simulink model "F16trim"  (R2013a)
settings: Solver=ode4  StartTime=0.0  StopTime=1  FixedStep=0.01  RelTol=1e-3
values from neighbouring files (symbols this model uses):
  airSpeed = 393.720000000000    (= 393.72)    [F16NolinearModelRemoveWindControlData_low.m]    (also in testdata.m)
  altitude = 9843    [F16Data.mat]    (also in F16LinmodTestData.m = trim_state(3); F16NolinearModelInitialData.m = trim_state(3); F16NolinearModelRemoveWindControlData_low.m; F16hi_7500_394_all.mat = 7500)
  b_ref = 9.144    [F16LinmodTestData.m]    (also in F16NolinearModelInitialData.m; F16NolinearModelRemoveWindControlData_low.m = 30; testdata.m = 30)
  beta = 0    [F16NolinearModelRemoveWindControlData_low.m]    (also in testdata.m)
  mass = 636.94*14.59428    (= 9295.6807032)    [F16LinmodTestData.m]    (also in F16NolinearModelInitialData.m; F16NolinearModelRemoveWindControlData_low.m = 636.94; testdata.m = 636.94)
  pqr = [0,0,0]    [F16NolinearModelRemoveWindControlData_low.m]    (also in testdata.m)
libraries: aerolibconvert2 x1, aerolibatmos2 x1, aerolibgravity2 x1, aerolibadyn x1
settings Model: Creator=Dai  LastModifiedBy=Dai

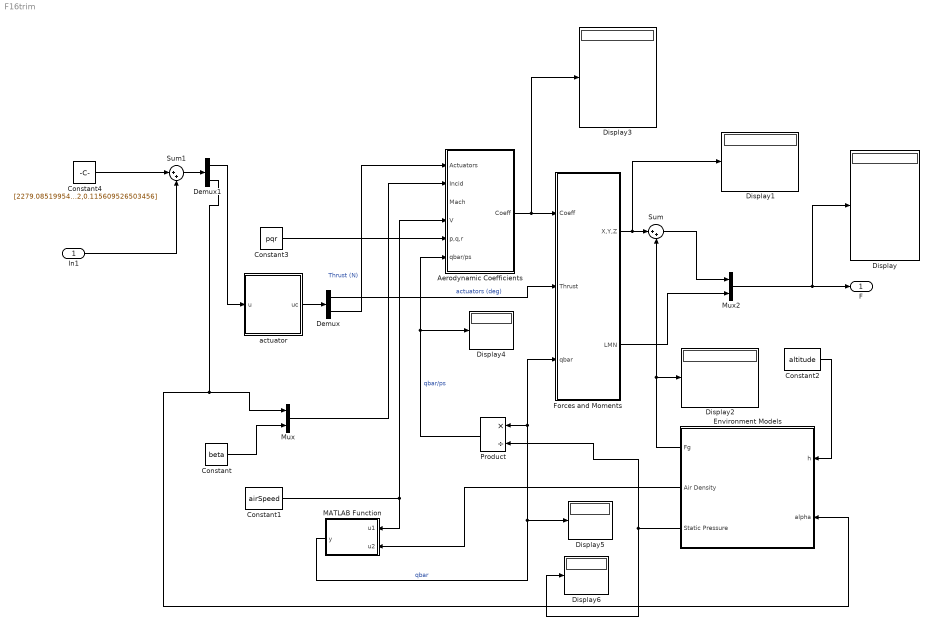
== system F16trim ==
  In1 : Inport  PortDimensions=5
  Aerodynamic Coefficients : Subsystem
  Constant : Constant  Value=beta
  Constant1 : Constant  Value=airSpeed
  Constant2 : Constant  Value=altitude
  Constant3 : Constant  Value=pqr
  Constant4 : Constant  Value=[2279.08519954656,-2.979731649,0.00874607850103852,0.0680302158182712,0.115609526503456]
  Demux : Demux  Outputs=2
  Demux1 : Demux  Outputs=[4,1]
  Display{,1..6} (7 alike) : Display
      Display settings: Decimation=6
      Display1 settings: Decimation=3
      Display2 settings: Decimation=3
      Display3 settings: Decimation=6
  Environment Models : Subsystem
  Forces and Moments : Subsystem
  MATLAB Function : MATLAB Function  TreatAsAtomicUnit=on
  Mux : Mux  Inputs=2
  Mux2 : Mux  Inputs=2
  Product : Product  Inputs=*/  SaturateOnIntegerOverflow=on  InputSameDT=on  OutDataTypeStr=Inherit: Same as first input
  Sum : Sum  Inputs=|++  SaturateOnIntegerOverflow=on  InputSameDT=on  OutDataTypeStr=Inherit: Same as first input
  Sum1 : Sum  Inputs=|++
  actuator : Subsystem
  F : Outport  PortDimensions=6
  wires:
  Aerodynamic Coefficients/1(Coeff) -> Display3/1, Forces and Moments/1(Coeff)
  Environment Models/2(Air Density) -> MATLAB Function/2(u2)
  Forces and Moments/2(LMN) -> Mux2/2
  MATLAB Function/1(y) -> Forces and Moments/3(qbar), Product/1, Display5/1  "qbar"
  Forces and Moments/1(X,Y,Z) -> Display1/1, Sum/1
  Environment Models/1(Fg) -> Display2/1, Sum/2
  Environment Models/3(Static Pressure) -> Display6/1, Product/2
  Product/1 -> Aerodynamic Coefficients/6(qbar/ps), Display4/1  "qbar/ps"
  actuator/1(uc) -> Demux/1
  Demux/1 -> Forces and Moments/2(Thrust)  "actuators (deg)"
  Demux/2 -> Aerodynamic Coefficients/1(Actuators)  "Thrust (N)"
  Demux1/2 -> Environment Models/2(alpha), Mux/1
  Constant/1 -> Mux/2
  Mux/1 -> Aerodynamic Coefficients/2(Incid)
  Constant1/1 -> MATLAB Function/1(u1), Aerodynamic Coefficients/4(V)
  Constant2/1 -> Environment Models/1(h)
  Constant3/1 -> Aerodynamic Coefficients/5(p,q,r)
  Demux1/1 -> actuator/1(u)
  Mux2/1 -> Display/1, F/1
  Constant4/1 -> Sum1/1
  Sum1/1 -> Demux1/1
  Sum/1 -> Mux2/1
  In1/1 -> Sum1/2

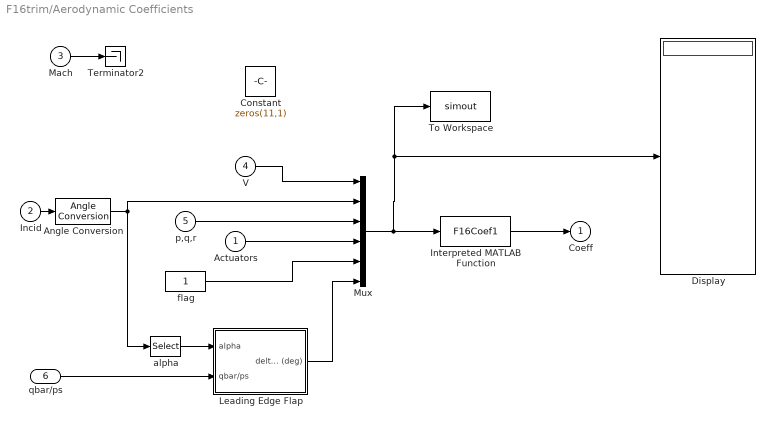
== system F16trim/Aerodynamic Coefficients ==
  Actuators : Inport
  Incid : Inport  Port=2
  Mach : Inport  Port=3
  V : Inport  Port=4
  p,q,r : Inport  Port=5
  qbar/ps : Inport  Port=6
  Angle Conversion : aerolibconvert2/Angle Conversion  IU=rad  OU=deg
  Constant : Constant  Value=zeros(11,1)
  Display : Display
      settings: Decimation=12
  Interpreted MATLAB Function : MATLABFcn  MATLABFcn=F16Coef1  OutputDimensions=6
  Leading Edge Flap : Subsystem
  Mux : Mux  Inputs=6
  Terminator2 : Terminator
  To Workspace : ToWorkspace  VariableName=simout  SampleTime=-1
  alpha : Selector  InputPortWidth=2  IndexOptions=Index vector (dialog)  Indices=1  OutputSizes=1
  flag : Constant
  Coeff : Outport  InitialOutput=0
  wires:
  Angle Conversion/1 -> alpha/1, Mux/2
  Incid/1 -> Angle Conversion/1
  qbar/ps/1 -> Leading Edge Flap/2(qbar/ps)
  alpha/1 -> Leading Edge Flap/1(alpha)
  V/1 -> Mux/1
  p,q,r/1 -> Mux/3
  Actuators/1 -> Mux/4
  flag/1 -> Mux/5
  Mach/1 -> Terminator2/1
  Interpreted MATLAB Function/1 -> Coeff/1
  Mux/1 -> To Workspace/1, Display/1, Interpreted MATLAB Function/1
  Leading Edge Flap/1(delta_lef (deg)) -> Mux/6

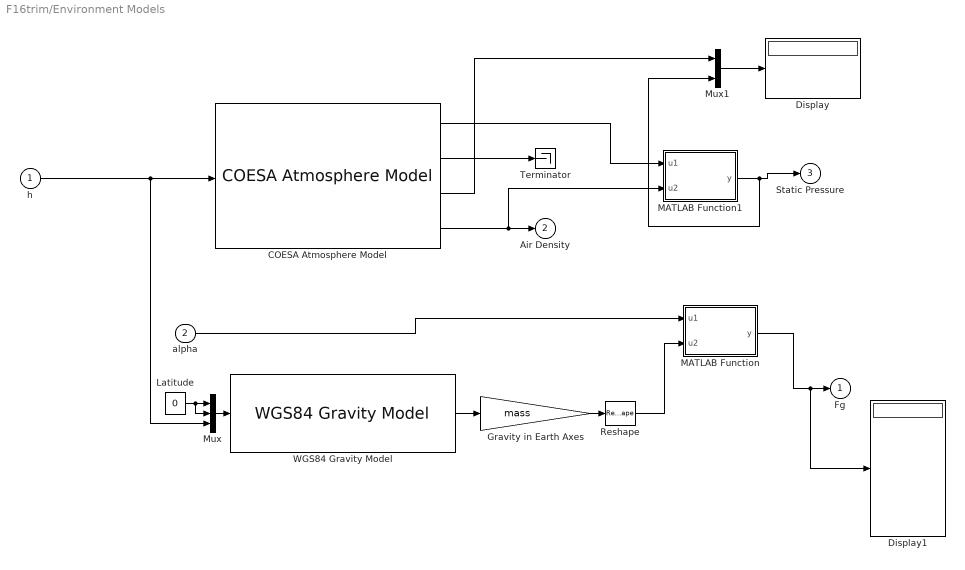
== system F16trim/Environment Models ==
  h : Inport  PortDimensions=1
  alpha : Inport  Port=2
  COESA Atmosphere Model : aerolibatmos2/COESA Atmosphere Model  units=English (Velocity in ft/s)  spec=1976 COESA-extended U.S. Standard Atmosphere  model=Profile  profile_var=High temperature  profile_percent=10%  profile_alt=5 km (16404 ft)  envelope_var=High temperature  envelope_percent=1%  action=None
  Display : Display
      settings: Decimation=2
  Display1 : Display
      settings: Decimation=3
  Gravity in Earth Axes : Gain  Gain=mass  SaturateOnIntegerOverflow=on  OutDataTypeStr=Inherit: Same as input  ParamDataTypeStr=Inherit: Same as input
  Latitude : Constant  Value=0
  MATLAB Function : MATLAB Function  TreatAsAtomicUnit=on
  MATLAB Function1 : MATLAB Function  TreatAsAtomicUnit=on
  Mux : Mux  Inputs=3
  Mux1 : Mux  Inputs=2
  Reshape : Reshape
  Terminator : Terminator
  "WGS84 Gravity Model " : aerolibgravity2/WGS84 Gravity Model   model=WGS84 Taylor Series  units=English  no_atmos=on  precessing=on  jd_loc=off  month=October  day=10  year=2004  no_centrifugal=on  action=None
  Fg : Outport  InitialOutput=0
  Air Density : Outport  Port=2  InitialOutput=0
  Static Pressure : Outport  Port=3
  wires:
  Reshape/1 -> MATLAB Function/2(u2)
  Mux/1 -> "WGS84 Gravity Model "/1
  h/1 -> Mux/3, COESA Atmosphere Model/1
  COESA Atmosphere Model/4 -> MATLAB Function1/2(u2), Air Density/1
  COESA Atmosphere Model/2 -> Terminator/1
  Latitude/1 -> Mux/2, Mux/1
  "WGS84 Gravity Model "/1 -> Gravity in Earth Axes/1
  Gravity in Earth Axes/1 -> Reshape/1
  alpha/1 -> MATLAB Function/1(u1)
  MATLAB Function/1(y) -> Display1/1, Fg/1
  COESA Atmosphere Model/1 -> MATLAB Function1/1(u1)
  MATLAB Function1/1(y) -> Mux1/2, Static Pressure/1
  COESA Atmosphere Model/3 -> Mux1/1
  Mux1/1 -> Display/1

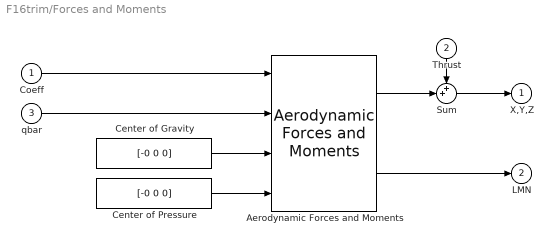
== system F16trim/Forces and Moments ==
  Coeff : Inport
  Thrust : Inport  Port=2
  qbar : Inport  Port=3
  "Aerodynamic Forces and Moments " : aerolibadyn/Aerodynamic Forces and Moments   inputAxes=Body  outputForceAxes=Body  outputMomentAxes=Body  S=S_ref  b=b_ref  cbar=d_ref
  Center of Gravity : Constant  Value=[-0 0 0]
  Center of Pressure : Constant  Value=[-0 0 0]
  Sum : Sum  Inputs=++|  SaturateOnIntegerOverflow=on  InputSameDT=on  OutDataTypeStr=Inherit: Same as first input
  X,Y,Z : Outport  InitialOutput=0
  LMN : Outport  Port=2  InitialOutput=0
  wires:
  Center of Pressure/1 -> "Aerodynamic Forces and Moments "/4
  Center of Gravity/1 -> "Aerodynamic Forces and Moments "/3
  "Aerodynamic Forces and Moments "/1 -> Sum/2
  "Aerodynamic Forces and Moments "/2 -> LMN/1
  Sum/1 -> X,Y,Z/1
  qbar/1 -> "Aerodynamic Forces and Moments "/2
  Coeff/1 -> "Aerodynamic Forces and Moments "/1
  Thrust/1 -> Sum/1

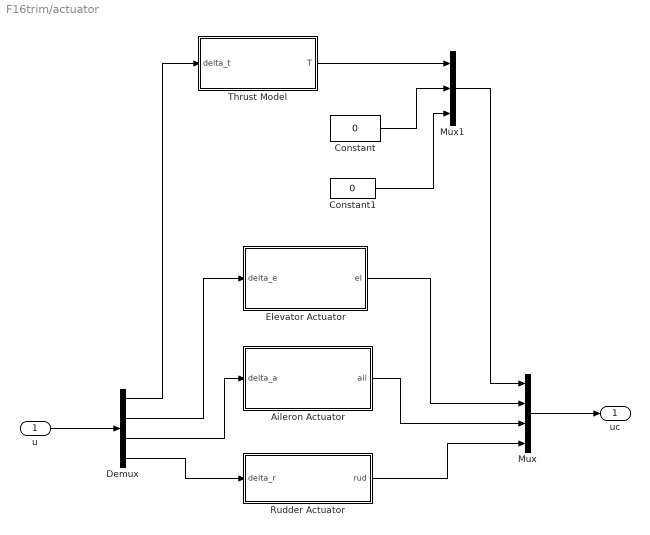
== system F16trim/actuator ==
  u : Inport
  Aileron Actuator : Subsystem
  Constant : Constant  Value=0
  Constant1 : Constant  Value=0
  Demux : Demux
  Elevator Actuator : Subsystem
  Mux : Mux
  Mux1 : Mux  Inputs=3
  Rudder Actuator : Subsystem
  Thrust Model : Subsystem
  uc : Outport
  wires:
  u/1 -> Demux/1
  Mux/1 -> uc/1
  Thrust Model/1(T) -> Mux1/1
  Constant/1 -> Mux1/2
  Constant1/1 -> Mux1/3
  Demux/1 -> Thrust Model/1(delta_t)
  Mux1/1 -> Mux/1
  Demux/2 -> Elevator Actuator/1(delta_e)
  Elevator Actuator/1(el) -> Mux/2
  Demux/3 -> Aileron Actuator/1(delta_a)
  Aileron Actuator/1(ail) -> Mux/3
  Demux/4 -> Rudder Actuator/1(delta_r)
  Rudder Actuator/1(rud) -> Mux/4

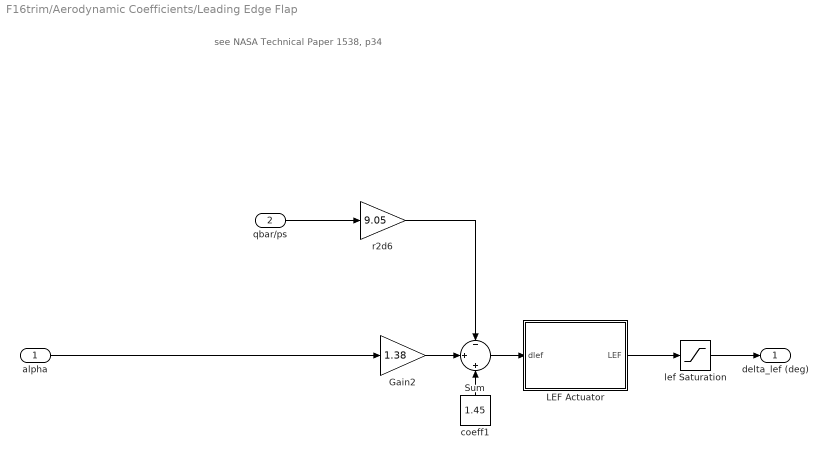
== system F16trim/Aerodynamic Coefficients/Leading Edge Flap ==
  note: see NASA Technical Paper 1538, p34
  alpha : Inport
  qbar/ps : Inport  Port=2
  Gain2 : Gain  Gain=1.38  SaturateOnIntegerOverflow=on  OutDataTypeStr=Inherit: Same as input  ParamDataTypeStr=Inherit: Same as input
  LEF Actuator : Subsystem
  Sum : Sum  Inputs=-|+|+  SaturateOnIntegerOverflow=on  InputSameDT=on  OutDataTypeStr=Inherit: Same as first input
  coeff1 : Constant  Value=1.45
  lef Saturation : Saturate  UpperLimit=25  LowerLimit=0
  r2d6 : Gain  Gain=9.05  SaturateOnIntegerOverflow=on  OutDataTypeStr=Inherit: Same as input  ParamDataTypeStr=Inherit: Same as input
  delta_lef (deg) : Outport
  wires:
  Gain2/1 -> Sum/2
  coeff1/1 -> Sum/3
  qbar/ps/1 -> r2d6/1
  r2d6/1 -> Sum/1
  lef Saturation/1 -> delta_lef (deg)/1
  Sum/1 -> LEF Actuator/1(dlef)
  LEF Actuator/1(LEF) -> lef Saturation/1
  alpha/1 -> Gain2/1

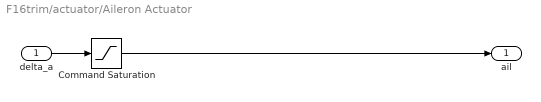
== system F16trim/actuator/Aileron Actuator ==
  delta_a : Inport
  Command Saturation : Saturate  UpperLimit=21.5  LowerLimit=-21.5
  ail : Outport
  wires:
  delta_a/1 -> Command Saturation/1
  Command Saturation/1 -> ail/1

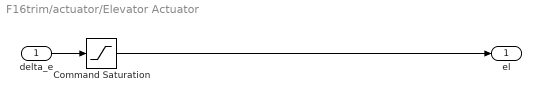
== system F16trim/actuator/Elevator Actuator ==
  delta_e : Inport
  Command Saturation : Saturate  UpperLimit=25  LowerLimit=-25
  el : Outport
  wires:
  delta_e/1 -> Command Saturation/1
  Command Saturation/1 -> el/1

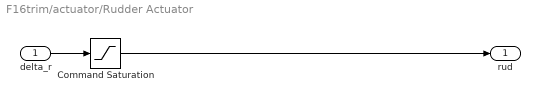
== system F16trim/actuator/Rudder Actuator ==
  delta_r : Inport
  Command Saturation : Saturate  UpperLimit=30  LowerLimit=-30
  rud : Outport
  wires:
  delta_r/1 -> Command Saturation/1
  Command Saturation/1 -> rud/1

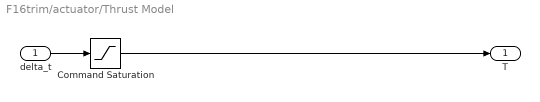
== system F16trim/actuator/Thrust Model ==
  delta_t : Inport
  Command Saturation : Saturate  UpperLimit=19000  LowerLimit=1000
  T : Outport
  wires:
  delta_t/1 -> Command Saturation/1
  Command Saturation/1 -> T/1

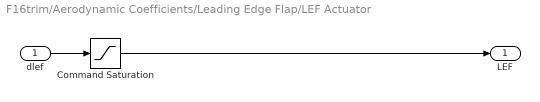
== system F16trim/Aerodynamic Coefficients/Leading Edge Flap/LEF Actuator ==
  dlef : Inport
  Command Saturation : Saturate  UpperLimit=25  LowerLimit=0
  LEF : Outport
  wires:
  dlef/1 -> Command Saturation/1
  Command Saturation/1 -> LEF/1

== matlab function F16trim/MATLAB Function ==
  data: u1 input; y output; u2 input
function y = fcn(u1,u2)
%#codegen

y = 0.5*u1^2*u2;

== matlab function F16trim/Environment Models/MATLAB Function ==
  data: u1 input; y output; u2 input
function y = fcn(u1,u2)
%#codegen
%u3=636.94*32.17;
y = [-u2(3)*sin(u1);0;u2(3)*cos(u1)];

== matlab function F16trim/Environment Models/MATLAB Function1 ==
  data: u1 input; y output; u2 input
function y = fcn(u1,u2)
%#codegen

y = 1715.0*u1*u2;
